simulink model "PitchSys"  (Simulink 9.0)
settings: Solver=ode1  StartTime=0.00  StopTime=50.00  FixedStep=0.01  RelTol=1e-3  EnableMultiTasking=on
undefined symbols (not defined in the file): Je, k_d, k_s, l1
settings Model: Creator=bjones  LastModifiedBy=Alex
settings DataIOCC: SignalLoggingSaveFormat=ModelDataLogs
settings OptimizationCC: BlockReduction=off  BooleanDataType=off  ExpressionDepthLimit=2147483647
settings DebuggingCC: SaveWithParameterizedLinksMsg=none  UnderspecifiedInitializationDetection=Simplified  MergeDetectMultiDrivingBlocksExec=error  SignalResolutionControl=TryResolveAllWithWarning  MultiTaskDSMMsg=warning  MultiTaskCondExecSysMsg=none  FcnCallInpInsideContextMsg=warning  StateNameClashWarn=warning  StrictBusMsg=None
settings HardwareCC: TargetUnknown=on
settings GRTTargetCC: GeneratePreprocessorConditionals=Disable all  CombineOutputUpdateFcns=off  GRTInterface=on
settings ConfigComp: CovSFcnEnable=off

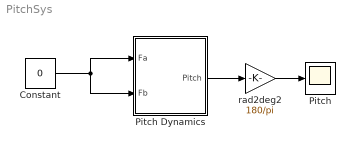
== system PitchSys ==
  Constant : Constant  Value=0
  Pitch : Scope
  Pitch Dynamics : Subsystem
  rad2deg2 : Gain  Gain=180/pi  SaturateOnIntegerOverflow=on  OutDataTypeStr=Inherit: Same as input  ParamDataTypeStr=Inherit: Same as input
  wires:
  Pitch Dynamics/1(Pitch) -> rad2deg2/1
  rad2deg2/1 -> Pitch/1
  Constant/1 -> Pitch Dynamics/1(Fa), Pitch Dynamics/2(Fb)

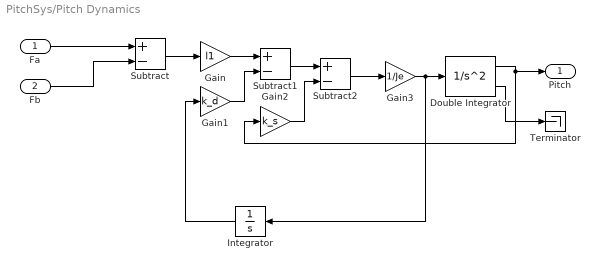
== system PitchSys/Pitch Dynamics ==
  Fa : Inport
  Fb : Inport  Port=2
  Double Integrator : SecondOrderIntegrator  ICX=p_lim_u  LimitX=on  UpperLimitX=p_lim_u  LowerLimitX=p_lim_l
  Gain : Gain  Gain=l1
  Gain1 : Gain  Gain=k_d
  Gain2 : Gain  Gain=k_s
  Gain3 : Gain  Gain=1/Je
  Integrator : Integrator
  Subtract : Sum  Inputs=+-
  Subtract1 : Sum  Inputs=+-
  Subtract2 : Sum  Inputs=+-
  Terminator : Terminator
  Pitch : Outport
  wires:
  Double Integrator/1 -> Gain2/1, Pitch/1
  Fa/1 -> Subtract/1
  Fb/1 -> Subtract/2
  Subtract/1 -> Gain/1
  Gain/1 -> Subtract1/1
  Gain1/1 -> Subtract1/2
  Subtract1/1 -> Subtract2/1
  Gain2/1 -> Subtract2/2
  Gain3/1 -> Integrator/1, Double Integrator/1
  Subtract2/1 -> Gain3/1
  Integrator/1 -> Gain1/1
  Double Integrator/2 -> Terminator/1
